simulink model "SR_EqnErr_Model"  (R2017b)
settings: Solver=ode5  StartTime=0.0  StopTime=15  FixedStep=0.025  RelTol=1e-3  EnableMultiTasking=on
values from neighbouring files (symbols this model uses):
  RGM3 = [-1 0 1 ... (first row only)    [setup.m]
undefined symbols (not defined in the file or in its folder): A1, B1
libraries: simulink x3
settings Model: Creator=b1048743  LastModifiedBy=Tom
settings DataIOCC: LimitDataPoints=on  SaveFormat=Array  SignalLoggingSaveFormat=ModelDataLogs  SignalLoggingName=sigsOut
settings OptimizationCC: BlockReduction=off  BooleanDataType=off
settings DebuggingCC: SaveWithParameterizedLinksMsg=none  UnderspecifiedInitializationDetection=Classic  MergeDetectMultiDrivingBlocksExec=none  SignalResolutionControl=TryResolveAllWithWarning  MultiTaskDSMMsg=warning  MultiTaskCondExecSysMsg=none
settings HardwareCC: ProdBitPerPointer=32  ProdBitPerSizeT=32  ProdBitPerPtrDiffT=32  ProdLargestAtomicFloat=None  ProdIntDivRoundTo=Undefined  ProdEndianess=Unspecified  ProdWordSize=32  ProdHWDeviceType=32-bit Generic  TargetUnknown=on
settings ModelReferenceCC: PropagateSignalLabelsOutOfModel=off
settings CodeAppCC: StateflowObjectComments=on
settings GRTTargetCC: TargetLangStandard=C89/C90 (ANSI)  CombineOutputUpdateFcns=off  GRTInterface=on
settings ConfigComp: CovMetricSettings=dw  CovHtmlReporting=on  CovSaveCumulativeToWorkspaceVar=on  CovSaveSingleToWorkspaceVar=on  CovExternalEMLEnable=off

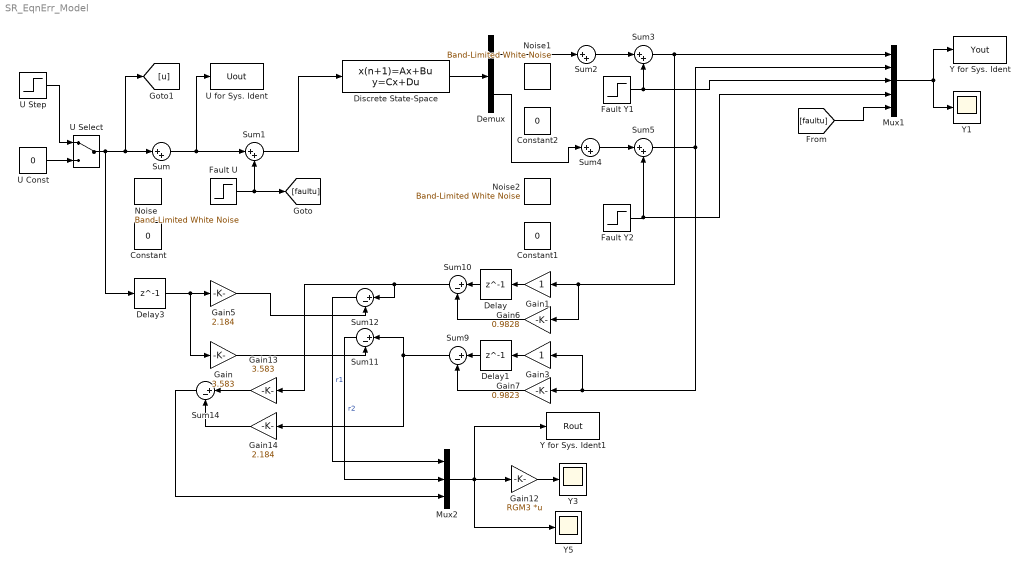
== system SR_EqnErr_Model ==
  Constant : Constant  Value=0
  Constant1 : Constant  Value=0
  Constant2 : Constant  Value=0
  Delay : Delay  DelayLength=1  SampleTime=0.025
  Delay1 : Delay  DelayLength=1  SampleTime=0.025
  Delay3 : Delay  DelayLength=1  SampleTime=0.025
  Demux : Demux  Outputs=2
  Discrete State-Space : DiscreteStateSpace  A=A1  B=B1  C=[1 0; 0 1]  D=[0;0]  SampleTime=0.025
  Fault U : Step  Time=5  After=0  SampleTime=0
  Fault Y1 : Step  Time=10  After=10  SampleTime=0
  Fault Y2 : Step  Time=10  After=0  SampleTime=0
  Gain : Gain  Gain=3.583
  Gain1 : Gain
  Gain12 : Gain  Gain=RGM3  Multiplication=Matrix(K*u)
  Gain13 : Gain  Gain=3.583
  Gain14 : Gain  Gain=2.184
  Gain3 : Gain
  Gain5 : Gain  Gain=2.184
  Gain6 : Gain  Gain=0.9828
  Gain7 : Gain  Gain=0.9823
  Mux1 : Mux  Inputs=5
  Mux2 : Mux  Inputs=3
  Noise : simulink/Sources/Band-Limited White Noise  Cov=[0.01]  Ts=0.025  seed=[23341]
  Noise1 : simulink/Sources/Band-Limited White Noise  Cov=[0.1]  Ts=0.025  seed=[23341]
  Noise2 : simulink/Sources/Band-Limited White Noise  Cov=[0.1]  Ts=0.025  seed=[23341]
  Sum{,1..5} (6 alike) : Sum  Inputs=|++  SaturateOnIntegerOverflow=on
  Sum{9..12,14} (5 alike) : Sum  Inputs=|+-
  U Const : Constant  Value=0
  "U Select " : ManualSwitch
  U Step : Step  SampleTime=0
  U for Sys. Ident : ToWorkspace  VariableName=Uout  SampleTime=0.025
  Y for Sys. Ident : ToWorkspace  VariableName=Yout  SampleTime=0.025
  Y for Sys. Ident1 : ToWorkspace  VariableName=Rout  SampleTime=0.025
  Y1 : Scope
  Y3 : Scope
  Y5 : Scope
  wires:
  U Const/1 -> "U Select "/2
  U Step/1 -> "U Select "/1
  Discrete State-Space/1 -> Demux/1
  Sum1/1 -> Discrete State-Space/1
  Fault U/1 -> [faultu], Sum1/2
  Sum2/1 -> Sum3/1
  Fault Y1/1 -> Sum3/2, Mux1/3
  Sum4/1 -> Sum5/1
  Fault Y2/1 -> Mux1/4, Sum5/2
  Demux/1 -> Sum2/1
  Demux/2 -> Sum4/1
  Sum/1 -> Sum1/1, U for Sys. Ident/1
  "U Select "/1 -> Delay3/1, [u], Sum/1
  Sum5/1 -> Gain3/1, Gain7/1, Mux1/2
  Sum12/1 -> Mux2/1  "r1"
  Gain1/1 -> Delay/1
  Gain3/1 -> Delay1/1
  Gain/1 -> Sum11/2
  Gain5/1 -> Sum12/2
  Delay3/1 -> Gain/1, Gain5/1
  Sum11/1 -> Mux2/2  "r2"
  Mux1/1 -> Y for Sys. Ident/1, Y1/1
  Sum10/1 -> Sum12/1, Gain13/1
  Gain6/1 -> Sum10/2
  Delay/1 -> Sum10/1
  Sum3/1 -> Mux1/1, Gain6/1, Gain1/1
  Delay1/1 -> Sum9/1
  Gain7/1 -> Sum9/2
  Sum9/1 -> Gain14/1, Sum11/1
  Gain12/1 -> Y3/1
  Gain13/1 -> Sum14/1
  Gain14/1 -> Sum14/2
  Sum14/1 -> Mux2/3
  Mux2/1 -> Y for Sys. Ident1/1, Y5/1, Gain12/1
  [faultu] -> Mux1/5
